simulink model "model_stanowisko"  (R2024a)
settings: Solver=VariableStepAuto  StartTime=0.0  StopTime=10.0  RelTol=1e-3
InitFcn:
  | a = 0.672; % M + ma/2 + mb, kg
  | b = 0.0051; % (ma/2 + mb)*L, kg*m
  | % c = 0.0021; % (ma/4 + mb)*L^2 + I, kg*m^2
  | g = 9.81;
  | u = 1;
  | 
  | T1 = 0.2;
  | T2 = 0.1;
  | Tf = 0.05;
  | 
  | x1 = 0;
  | x2 = 0;
  | x3 = 0;
  | x4 = 0;
  | x1p = 0;
  | x2p = 0;
  | x3p = 0;
  | x4p = 0;
  | 
  | r = 1;
  | 
  | b0 = 1;
  | A = [0 1 0;
  |      0 0 1;
  |      0 0 0];
  | b_ = [0; b0; 0];
  | c = [1; 0; 0];
  | 
  | % A_CP = [0 1;
  | %        0 0];
  | %
  | % b_CP = [0; 1];
  | %
  | % w_CL = 70;
  | %
  | % k = place(A_CP', b_CP, -w_CL*[1 1.01])';
  | %
  | % k_ESO = 0.9;
  | %
  | % l = place(A',c,-w_CL*k_ESO*[0.99,1,1.01])';
  | 
  | % k_ESO = 10;
  | 
  | % wc_ = 70;
  | % Kx_ = place(A',b_,-wc_*[1 1])';
  | %
  | % k = [5;5];
  | %
  | % w0 = 60;
  | % l = place(A',c,-w0*[0.99,1,1.01])';
  | 
  | %% Liczenie k
  | w_CL = 5;
  | n=2;
  | k = zeros(n,1);
  | for i = 1:n
  |     k(i) = ((factorial(n))/(factorial(n-i+1)*factorial(i-1)))*w_CL^(n-i+1);
  | end
  | 
  | k_r = [k(2); 1];
  | 
  | %% Liczenie l
  | k_ESO = 50;
  | l = zeros(n+1,1);
  | 
  | for i = 1:n+1
  |     l(i) = (factorial(n+1)/(factorial(n-i+1)*factorial(i)))*(k_ESO)^(i);
  | end
  | 
  | % %% PRZYPISANIE POSZCZEGÓLNYCH L:
  | % l1 = l(1);
  | % l2 = l(2);
  | % %% OKREŚLENIE BETY:
  | % B1 = 3 * k_ESO;
  | % B2 = 3 * k_ESO^2;
  | % B3 = k_ESO^3;
  | 
  | %% W ARTYKULE MADONSKI K,L ODPOWIADA L I B W ARTYKULE JIN H.
  | l1 = k(2);
  | l2 = k(1);
  | 
  | B1 = l(1);
  | B2 = l(2);
  | B3 = l(3);
  | 
  | %% WYZNACZENIE PARAMETRÓW:
  | Kc = (B2 * l2 + B3 * l1)/(b0*(B1 * l1 + B2 + l2));
  | tau_i = (B2 * l2 + B3 * l1)/(B3 * l2);
  | tau_d = (B1 * l2 + B2 * l1 + B3)/(B2 * l2 + B3 * l1);
  | wl = sqrt(B1 * l1 + B2 + l2);
  | zeta_l = (B1 + l1)/(2*sqrt(B1 * l1 + B2 + l2));
  | %% Wzmocnienia regulatora CPID:
  | Kp = Kc;
  | Ki = Kc/tau_i;
  | Kd = Kc * tau_d;
  | 
  | %% NOWE NASTAWY PID
  | % Kp = (k(1)*l(1)+k(2)*l(3))/(b0*(k(2)*l(1)+l(2)+k(1)));
  | % Ki = (k(1)*l(3))/(b0*(k(2)*l(1)+l(2)+k(1)));
  | % Kd = (k(1)*l(1)+k(2)*l(2)+l(3))/(b0*(k(2)*l(1)+l(2)+k(1)));
libraries: simulink x2
settings Model: Creator=kubat  LastModifiedBy=kubat

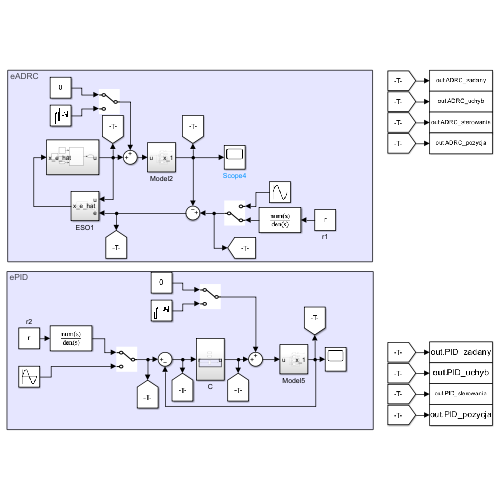
[thumbnail: Simulink's stored preview of the top-level diagram]
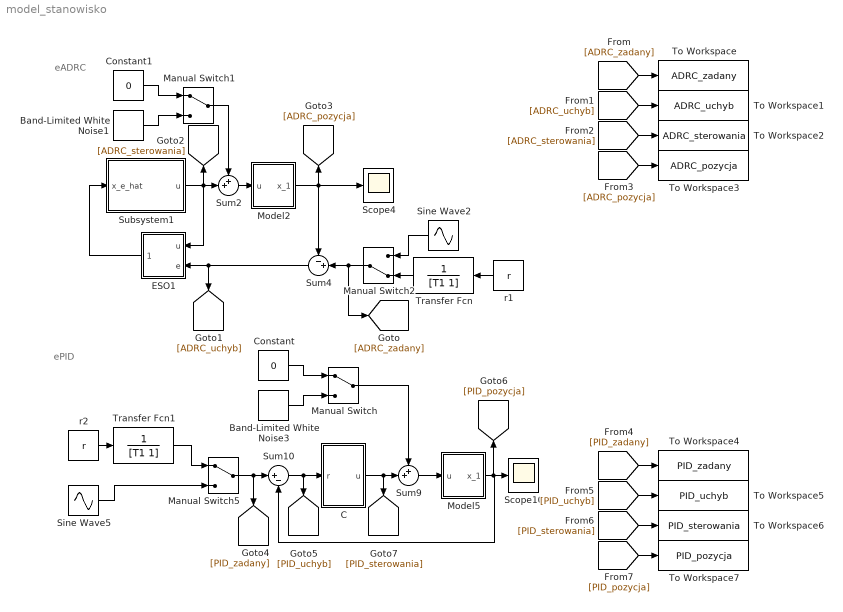
== system model_stanowisko ==
  note: ePID
  note: eADRC
  Band-Limited White Noise1 : simulink/Sources/Band-Limited White Noise  Cov=[0.001]  Ts=0.01  seed=[23341]
  Band-Limited White Noise3 : simulink/Sources/Band-Limited White Noise  Cov=[0.001]  Ts=0.01  seed=[23341]
  C : Subsystem
  Constant : Constant  Value=0
  Constant1 : Constant  Value=0
  ESO1 : Subsystem
  Manual Switch : ManualSwitch
  Manual Switch1 : ManualSwitch
  Manual Switch2 : ManualSwitch  CurrentSetting=0
  Manual Switch5 : ManualSwitch
  Model2 : Subsystem
  Model5 : Subsystem
  Scope10 : Scope
  Scope4 : Scope
  Sine Wave2 : Sin  Amplitude=u  SampleTime=0
  Sine Wave5 : Sin  Amplitude=u  SampleTime=0
  Subsystem1 : Subsystem
  Sum10 : Sum  Inputs=|+-
  Sum2 : Sum  Inputs=++|
  Sum4 : Sum  Inputs=-+|
  Sum9 : Sum  Inputs=++|
  To Workspace : ToWorkspace  VariableName=ADRC_zadany  SaveFormat=Timeseries  SampleTime=-1
  To Workspace1 : ToWorkspace  VariableName=ADRC_uchyb  SaveFormat=Timeseries  SampleTime=-1
  To Workspace2 : ToWorkspace  VariableName=ADRC_sterowania  SaveFormat=Timeseries  SampleTime=-1
  To Workspace3 : ToWorkspace  VariableName=ADRC_pozycja  SaveFormat=Timeseries  SampleTime=-1
  To Workspace4 : ToWorkspace  VariableName=PID_zadany  SaveFormat=Timeseries  SampleTime=-1
  To Workspace5 : ToWorkspace  VariableName=PID_uchyb  SaveFormat=Timeseries  SampleTime=-1
  To Workspace6 : ToWorkspace  VariableName=PID_sterowania  SaveFormat=Timeseries  SampleTime=-1
  To Workspace7 : ToWorkspace  VariableName=PID_pozycja  SaveFormat=Timeseries  SampleTime=-1
  Transfer Fcn : TransferFcn  Denominator=[T1 1]
  Transfer Fcn1 : TransferFcn  Denominator=[T1 1]
  r1 : Constant  Value=r
  r2 : Constant  Value=r
  wires:
  Sum2/1 -> Model2/1(u)
  ESO1/1(x_e_hat) -> Subsystem1/1(x_e_hat)
  Model5/1(x_1) -> [PID_pozycja], Sum10/2, Scope10/1
  Sum9/1 -> Model5/1(u)
  Manual Switch2/1 -> [ADRC_zadany], Sum4/2
  Model2/1(x_1) -> Sum4/1, Scope4/1, [ADRC_pozycja]
  Subsystem1/1(u) -> [ADRC_sterowania], ESO1/1(u), Sum2/2
  Sum10/1 -> [PID_uchyb], C/1(r)
  Manual Switch5/1 -> [PID_zadany], Sum10/1
  Transfer Fcn1/1 -> Manual Switch5/1
  r2/1 -> Transfer Fcn1/1
  Sine Wave5/1 -> Manual Switch5/2
  r1/1 -> Transfer Fcn/1
  Sum4/1 -> [ADRC_uchyb], ESO1/2(e)
  C/1(u) -> [PID_sterowania], Sum9/2
  Transfer Fcn/1 -> Manual Switch2/2
  Sine Wave2/1 -> Manual Switch2/1
  Band-Limited White Noise3/1 -> Manual Switch/2
  Manual Switch/1 -> Sum9/1
  Constant/1 -> Manual Switch/1
  Constant1/1 -> Manual Switch1/1
  Band-Limited White Noise1/1 -> Manual Switch1/2
  Manual Switch1/1 -> Sum2/1
  [ADRC_zadany] -> To Workspace/1
  [ADRC_uchyb] -> To Workspace1/1
  [ADRC_sterowania] -> To Workspace2/1
  [ADRC_pozycja] -> To Workspace3/1
  [PID_pozycja] -> To Workspace7/1
  [PID_sterowania] -> To Workspace6/1
  [PID_uchyb] -> To Workspace5/1
  [PID_zadany] -> To Workspace4/1

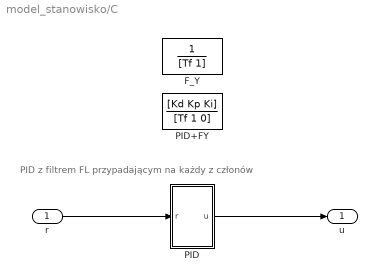
== system model_stanowisko/C ==
  note: PID z filtrem FL przypadającym na każdy z członów
  r : Inport
  F_Y : TransferFcn  Denominator=[Tf 1]
  PID : Subsystem
  PID+FY : TransferFcn  Numerator=[Kd Kp Ki]  Denominator=[Tf 1 0]
  u : Outport
  wires:
  r/1 -> PID/1(r)
  PID/1(u) -> u/1

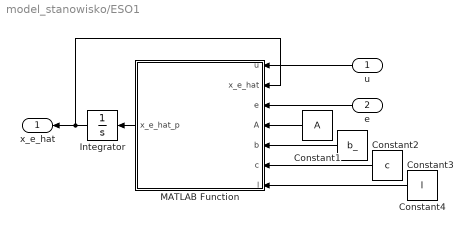
== system model_stanowisko/ESO1 ==
  u : Inport
  e : Inport  Port=2
  Constant1 : Constant  Value=A
  Constant2 : Constant  Value=b_
  Constant3 : Constant  Value=c
  Constant4 : Constant  Value=l
  Integrator : Integrator
  MATLAB Function : MATLAB Function  TreatAsAtomicUnit=on
  x_e_hat : Outport
  wires:
  Constant3/1 -> MATLAB Function/6(c)
  Integrator/1 -> x_e_hat/1, MATLAB Function/2(x_e_hat)
  MATLAB Function/1(x_e_hat_p) -> Integrator/1
  Constant2/1 -> MATLAB Function/5(b)
  e/1 -> MATLAB Function/3(e)
  Constant1/1 -> MATLAB Function/4(A)
  Constant4/1 -> MATLAB Function/7(l)
  u/1 -> MATLAB Function/1(u)

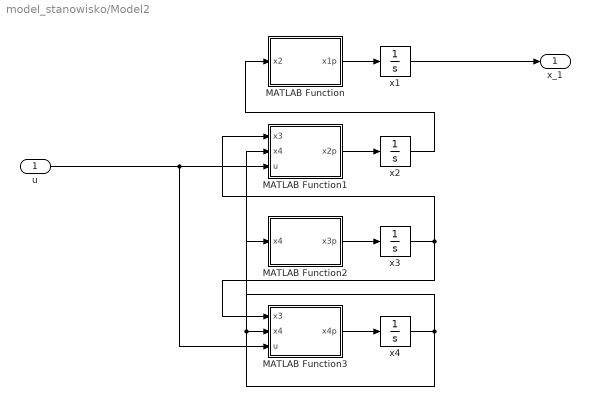
== system model_stanowisko/Model2 ==
  u : Inport
  MATLAB Function : MATLAB Function  TreatAsAtomicUnit=on
  MATLAB Function1 : MATLAB Function  TreatAsAtomicUnit=on
  MATLAB Function2 : MATLAB Function  TreatAsAtomicUnit=on
  MATLAB Function3 : MATLAB Function  TreatAsAtomicUnit=on
  x{1..4} (4 alike) : Integrator
  x_1 : Outport
  wires:
  u/1 -> MATLAB Function3/3(u), MATLAB Function1/3(u)
  x4/1 -> MATLAB Function2/1(x4), MATLAB Function3/2(x4), MATLAB Function1/2(x4)
  MATLAB Function/1(x1p) -> x1/1
  x3/1 -> MATLAB Function1/1(x3), MATLAB Function3/1(x3)
  x2/1 -> MATLAB Function/1(x2)
  MATLAB Function2/1(x3p) -> x3/1
  MATLAB Function1/1(x2p) -> x2/1
  MATLAB Function3/1(x4p) -> x4/1
  x1/1 -> x_1/1

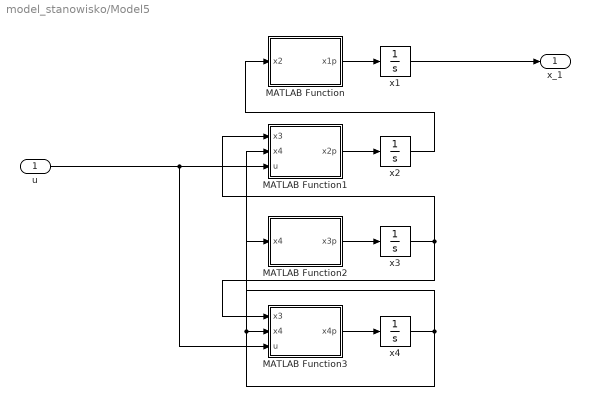
== system model_stanowisko/Model5 ==
  u : Inport
  MATLAB Function : MATLAB Function  TreatAsAtomicUnit=on
  MATLAB Function1 : MATLAB Function  TreatAsAtomicUnit=on
  MATLAB Function2 : MATLAB Function  TreatAsAtomicUnit=on
  MATLAB Function3 : MATLAB Function  TreatAsAtomicUnit=on
  x{1..4} (4 alike) : Integrator
  x_1 : Outport
  wires:
  u/1 -> MATLAB Function3/3(u), MATLAB Function1/3(u)
  x4/1 -> MATLAB Function3/2(x4), MATLAB Function1/2(x4), MATLAB Function2/1(x4)
  MATLAB Function/1(x1p) -> x1/1
  x3/1 -> MATLAB Function1/1(x3), MATLAB Function3/1(x3)
  x2/1 -> MATLAB Function/1(x2)
  MATLAB Function2/1(x3p) -> x3/1
  MATLAB Function1/1(x2p) -> x2/1
  MATLAB Function3/1(x4p) -> x4/1
  x1/1 -> x_1/1

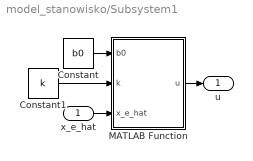
== system model_stanowisko/Subsystem1 ==
  x_e_hat : Inport
  Constant : Constant  Value=b0
  Constant1 : Constant  Value=k
  MATLAB Function : MATLAB Function  TreatAsAtomicUnit=on
  u : Outport
  wires:
  Constant/1 -> MATLAB Function/1(b0)
  Constant1/1 -> MATLAB Function/2(k)
  x_e_hat/1 -> MATLAB Function/3(x_e_hat)
  MATLAB Function/1(u) -> u/1

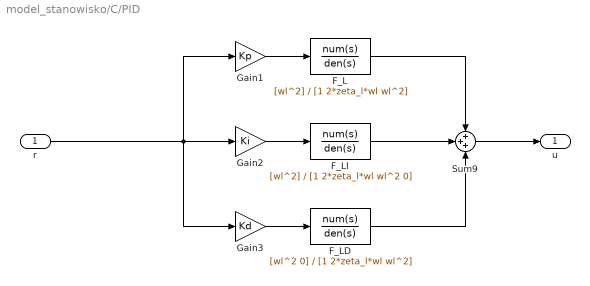
== system model_stanowisko/C/PID ==
  r : Inport
  F_L : TransferFcn  Numerator=[wl^2]  Denominator=[1 2*zeta_l*wl wl^2]
  F_LD : TransferFcn  Numerator=[wl^2 0]  Denominator=[1 2*zeta_l*wl wl^2]
  F_LI : TransferFcn  Numerator=[wl^2]  Denominator=[1 2*zeta_l*wl wl^2 0]
  Gain1 : Gain  Gain=Kp
  Gain2 : Gain  Gain=Ki
  Gain3 : Gain  Gain=Kd
  Sum9 : Sum  Inputs=+++
  u : Outport
  wires:
  Gain1/1 -> F_L/1
  r/1 -> Gain3/1, Gain2/1, Gain1/1
  Sum9/1 -> u/1
  F_L/1 -> Sum9/1
  Gain2/1 -> F_LI/1
  F_LI/1 -> Sum9/2
  Gain3/1 -> F_LD/1
  F_LD/1 -> Sum9/3

== matlab function model_stanowisko/ESO1/MATLAB Function ==
  data: u input; x_e_hat_p output; x_e_hat input; e input; A input; b input; c input; l input
function x_e_hat_p = fcn(u, x_e_hat, e, A, b, c, l)
c = c.';
pom1 = c*x_e_hat;
pom2 = e - pom1;

x_e_hat_p1 = A*x_e_hat-b*u+l*pom2;
x_e_hat_p = x_e_hat_p1(:,1);

== matlab function model_stanowisko/Model2/MATLAB Function ==
  data: x2 input; x1p output
function x1p = fcn(x2)

x1p = x2;

== matlab function model_stanowisko/Model2/MATLAB Function1 ==
  data: x3 input; x2p output; x4 input; u input
function x2p = fcn(x3, x4,u)
g = 9.81;
x2p = ((0.0031*u)/(0.0021-0.000038*cos(x3)^2))-(0.000016*sin(x3)*x4^2+0.000038*g*sin(x3)*cos(x3))/(0.0021-0.000038*cos(x3)^2);

== matlab function model_stanowisko/Model2/MATLAB Function2 ==
  data: x4 input; x3p output
function x3p = fcn(x4)

x3p = x4;

== matlab function model_stanowisko/Model2/MATLAB Function3 ==
  data: x3 input; x4 input; x4p output; u input
function x4p = fcn(x3,x4,u)
g = 9.81;
x4p = ((-0.0076*cos(x3)*u)/(0.0021-0.000038*cos(x3)^2))+(((-0.000038*sin(x3)*cos(x3)*x4^2) + 0.0051*g*sin(x3))/(0.0021-0.000038*cos(x3)^2));

== matlab function model_stanowisko/Subsystem1/MATLAB Function ==
  data: b0 input; u output; k input; x_e_hat input
function u = fcn(b0, k, x_e_hat)

k = k';
kpom = [k, 1];
b0_1 = 1/b0;
u = b0_1*(kpom*x_e_hat);

== matlab function model_stanowisko/Model5/MATLAB Function ==
  data: x2 input; x1p output
function x1p = fcn(x2)

x1p = x2;

== matlab function model_stanowisko/Model5/MATLAB Function1 ==
  data: x3 input; x2p output; x4 input; u input
function x2p = fcn(x3, x4,u)
g = 9.81;
x2p = ((0.0031*u)/(0.0021-0.000038*cos(x3)^2))-(0.000016*sin(x3)*x4^2+0.000038*g*sin(x3)*cos(x3))/(0.0021-0.000038*cos(x3)^2);

== matlab function model_stanowisko/Model5/MATLAB Function2 ==
  data: x4 input; x3p output
function x3p = fcn(x4)

x3p = x4;

== matlab function model_stanowisko/Model5/MATLAB Function3 ==
  data: x3 input; x4 input; x4p output; u input
function x4p = fcn(x3,x4,u)
g = 9.81;
x4p = ((-0.0076*cos(x3)*u)/(0.0021-0.000038*cos(x3)^2))+(((-0.000038*sin(x3)*cos(x3)*x4^2) + 0.0051*g*sin(x3))/(0.0021-0.000038*cos(x3)^2));
